simulink model "EurlerDynJointVerify"  (Simulink 7.6)
settings: Solver=ode45  StartTime=0.0  StopTime=10  RelTol=1e-3
InitFcn:
  | eval('Config')
  | %eval('EfortConfig')
values from neighbouring files (symbols this model uses):
  a2 = 0    [Config.m]    (also in CtrPlatformCfg.m)
  a3 = 0    [Config.m]    (also in CtrPlatformCfg.m)
  a4 = 0    [Config.m]    (also in CtrPlatformCfg.m)
  a5 = 90    [Config.m]    (also in CtrPlatformCfg.m)
  a6 = 0    [Config.m]    (also in CtrPlatformCfg.m)
  Cen_EU = Cen    [DynEulerTest.m]
  DH_EU = [266     300     0       0       1016     0      174 ... (first row only)    [DynEulerTest.m]
  freq = tvel/radius    (= 1)    [Config.m]    (also in CtrPlatformCfg.m)
  Ft_EU = [0;0;0;0;0;0]    [DynEulerTest.m]
  Ie_EU = [Ie1;Ie2;Ie3;Ie4;Ie5;Ie6]    [DynEulerTest.m]
  init_Endx = gd_init(1,4)    [Config.m]    (also in CtrPlatformCfg.m)
  init_Endy = gd_init(2,4)    [Config.m]    (also in CtrPlatformCfg.m)
  init_Endz = gd_init(3,4)    [Config.m]    (also in CtrPlatformCfg.m)
  init_Rot = gd_init(1:3,1:3)    [Config.m]    (also in CtrPlatformCfg.m)
  L = [l1 l2 l3 l4 l5 l6 l7 l8 l9]    [Config.m]    (also in CtrPlatformCfg.m)
  Ma_EU = Ma    [DynEulerTest.m]
  tvel = 120    [Config.m]    (also in CtrPlatformCfg.m)
undefined symbols (not defined in the file or in its folder): a1, Cen_Min, DH_Min, Ft_Min, Ie_Min, Ma_Min
libraries: mblibv1 x41, simulink x9
(part 3 of 3)

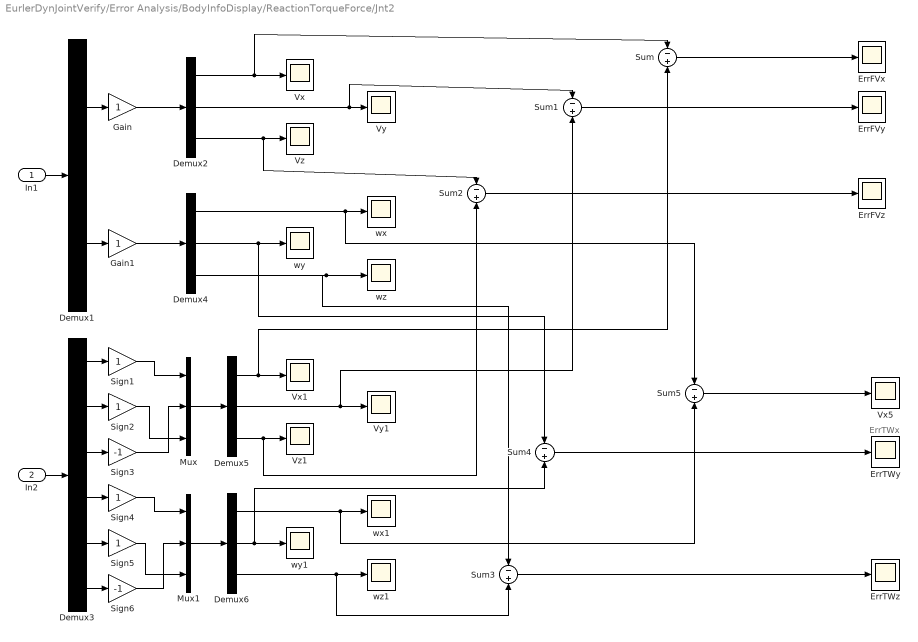
== system EurlerDynJointVerify/Error Analysis/BodyInfoDisplay/ReactionTorqueForce/Jnt2 ==
  note: ErrTWx
  In1 : Inport
  In2 : Inport  Port=2
  Demux1 : Demux  Outputs=2
  Demux{2,4..6} (4 alike) : Demux  Outputs=3
  Demux3 : Demux  Outputs=6
  ErrFVx : Scope
      settings: TimeRange=10  YMin=-3e-017  YMax=4e-017  SaveName=ScopeData51
  ErrFVy : Scope
      settings: TimeRange=10  YMin=-3e-017  YMax=4e-017  SaveName=ScopeData52
  ErrFVz : Scope
      settings: TimeRange=10  YMin=-3e-017  YMax=4e-017  SaveName=ScopeData53
  ErrTWy : Scope
      settings: TimeRange=10  YMin=-3e-017  YMax=4e-017  SaveName=ScopeData56
  ErrTWz : Scope
      settings: TimeRange=3  YMin=-1.5e-014  YMax=1.5e-014  SaveName=ScopeData68
  Gain : Gain
  Gain1 : Gain
  Mux : Mux  Inputs=3
  Mux1 : Mux  Inputs=3
  Sign{1..2,4..5} (4 alike) : Gain
  Sign3 : Gain  Gain=-1
  Sign6 : Gain  Gain=-1
  Sum{,1..5} (6 alike) : Sum  Inputs=-|+
  Vx : Scope
      settings: TimeRange=10  YMin=-3e-017  YMax=4e-017  SaveName=ScopeData40
  Vx1 : Scope
      settings: TimeRange=10  YMin=-3e-017  YMax=4e-017  SaveName=ScopeData45
  Vx5 : Scope
      settings: TimeRange=10  YMin=-3e-017  YMax=4e-017  SaveName=ScopeData54
  Vy : Scope
      settings: TimeRange=10  YMin=-3e-017  YMax=4e-017  SaveName=ScopeData39
  Vy1 : Scope
      settings: TimeRange=10  YMin=-3e-017  YMax=4e-017  SaveName=ScopeData46
  Vz : Scope
      settings: TimeRange=10  YMin=-3e-017  YMax=4e-017  SaveName=ScopeData41
  Vz1 : Scope
      settings: TimeRange=10  YMin=-3e-017  YMax=4e-017  SaveName=ScopeData47
  wx : Scope
      settings: TimeRange=3  YMin=-125  YMax=125  SaveName=ScopeData42
  wx1 : Scope
      settings: TimeRange=3  YMin=-125  YMax=125  SaveName=ScopeData48
  wy : Scope
      settings: TimeRange=10  YMin=-3e-017  YMax=4e-017  SaveName=ScopeData43
  wy1 : Scope
      settings: TimeRange=10  YMin=-3e-017  YMax=4e-017  SaveName=ScopeData49
  wz : Scope
      settings: TimeRange=10  YMin=-3e-017  YMax=4e-017  SaveName=ScopeData44
  wz1 : Scope
      settings: TimeRange=10  YMin=-3e-017  YMax=4e-017  SaveName=ScopeData50
  wires:
  Sign4/1 -> Mux1/1
  Sign1/1 -> Mux/1
  Demux3/6 -> Sign6/1
  Demux3/5 -> Sign5/1
  Demux3/4 -> Sign4/1
  Demux3/3 -> Sign3/1
  Demux3/2 -> Sign2/1
  Demux3/1 -> Sign1/1
  Mux1/1 -> Demux6/1
  Mux/1 -> Demux5/1
  Sum/1 -> ErrFVx/1
  Sum1/1 -> ErrFVy/1
  Sum2/1 -> ErrFVz/1
  Sum3/1 -> ErrTWz/1
  Sum4/1 -> ErrTWy/1
  Sum5/1 -> Vx5/1
  In2/1 -> Demux3/1
  Demux6/3 -> Sum3/2, wz1/1
  Demux6/2 -> Sum4/2, wy1/1
  Demux6/1 -> Sum5/2, wx1/1
  Demux5/3 -> Sum2/2, Vz1/1
  Demux5/2 -> Sum1/2, Vy1/1
  Demux5/1 -> Sum/2, Vx1/1
  In1/1 -> Demux1/1
  Demux4/3 -> Sum3/1, wz/1
  Demux4/2 -> Sum4/1, wy/1
  Demux4/1 -> Sum5/1, wx/1
  Demux2/3 -> Sum2/1, Vz/1
  Demux2/2 -> Sum1/1, Vy/1
  Demux2/1 -> Sum/1, Vx/1
  Gain1/1 -> Demux4/1
  Gain/1 -> Demux2/1
  Demux1/2 -> Gain1/1
  Demux1/1 -> Gain/1
  Sign3/1 -> Mux/2
  Sign2/1 -> Mux/3
  Sign6/1 -> Mux1/2
  Sign5/1 -> Mux1/3

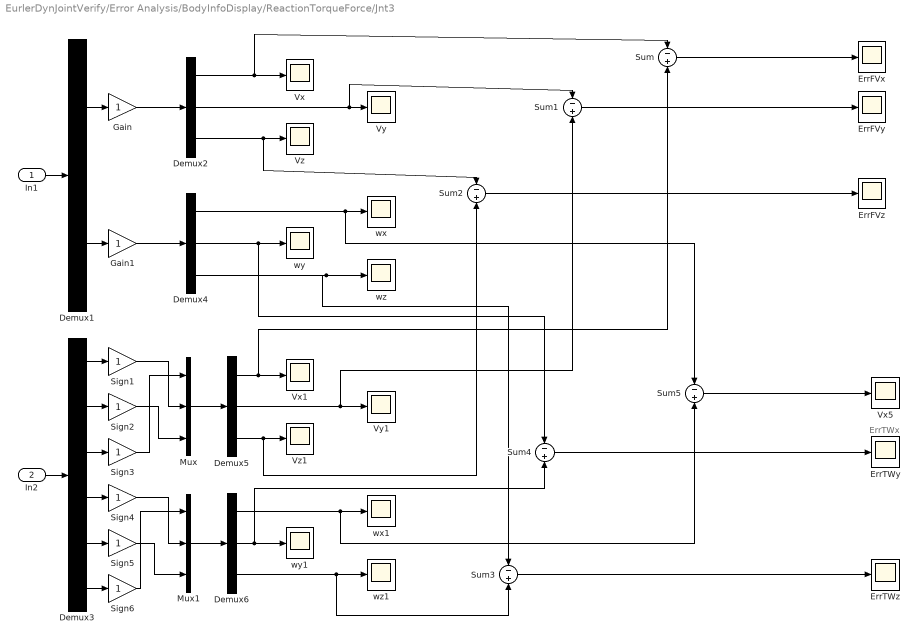
== system EurlerDynJointVerify/Error Analysis/BodyInfoDisplay/ReactionTorqueForce/Jnt3 ==
  note: ErrTWx
  In1 : Inport
  In2 : Inport  Port=2
  Demux1 : Demux  Outputs=2
  Demux{2,4..6} (4 alike) : Demux  Outputs=3
  Demux3 : Demux  Outputs=6
  ErrFVx : Scope
      settings: TimeRange=10  YMin=-3e-017  YMax=4e-017  SaveName=ScopeData51
  ErrFVy : Scope
      settings: TimeRange=10  YMin=-3e-017  YMax=4e-017  SaveName=ScopeData52
  ErrFVz : Scope
      settings: TimeRange=10  YMin=-3e-017  YMax=4e-017  SaveName=ScopeData53
  ErrTWy : Scope
      settings: TimeRange=10  YMin=-3e-017  YMax=4e-017  SaveName=ScopeData56
  ErrTWz : Scope
      settings: TimeRange=10  YMin=-3e-017  YMax=4e-017  SaveName=ScopeData68
  Gain : Gain
  Gain1 : Gain
  Mux : Mux  Inputs=3
  Mux1 : Mux  Inputs=3
  Sign{1..6} (6 alike) : Gain
  Sum{,1..5} (6 alike) : Sum  Inputs=-|+
  Vx : Scope
      settings: TimeRange=10  YMin=-3e-017  YMax=4e-017  SaveName=ScopeData40
  Vx1 : Scope
      settings: TimeRange=10  YMin=-3e-017  YMax=4e-017  SaveName=ScopeData45
  Vx5 : Scope
      settings: TimeRange=10  YMin=-3e-017  YMax=4e-017  SaveName=ScopeData54
  Vy : Scope
      settings: TimeRange=10  YMin=-3e-017  YMax=4e-017  SaveName=ScopeData39
  Vy1 : Scope
      settings: TimeRange=10  YMin=-3e-017  YMax=4e-017  SaveName=ScopeData46
  Vz : Scope
      settings: TimeRange=10  YMin=-3e-017  YMax=4e-017  SaveName=ScopeData41
  Vz1 : Scope
      settings: TimeRange=10  YMin=-3e-017  YMax=4e-017  SaveName=ScopeData47
  wx : Scope
      settings: TimeRange=3  YMin=-125  YMax=125  SaveName=ScopeData42
  wx1 : Scope
      settings: TimeRange=3  YMin=-125  YMax=125  SaveName=ScopeData48
  wy : Scope
      settings: TimeRange=10  YMin=-3e-017  YMax=4e-017  SaveName=ScopeData43
  wy1 : Scope
      settings: TimeRange=10  YMin=-3e-017  YMax=4e-017  SaveName=ScopeData49
  wz : Scope
      settings: TimeRange=10  YMin=-3e-017  YMax=4e-017  SaveName=ScopeData44
  wz1 : Scope
      settings: TimeRange=10  YMin=-3e-017  YMax=4e-017  SaveName=ScopeData50
  wires:
  Demux1/1 -> Gain/1
  Demux1/2 -> Gain1/1
  Gain/1 -> Demux2/1
  Gain1/1 -> Demux4/1
  Demux2/1 -> Vx/1, Sum/1
  Demux2/2 -> Vy/1, Sum1/1
  Demux2/3 -> Vz/1, Sum2/1
  Demux4/1 -> wx/1, Sum5/1
  Demux4/2 -> wy/1, Sum4/1
  Demux4/3 -> wz/1, Sum3/1
  In1/1 -> Demux1/1
  Demux5/1 -> Vx1/1, Sum/2
  Demux5/2 -> Vy1/1, Sum1/2
  Demux5/3 -> Vz1/1, Sum2/2
  Demux6/1 -> wx1/1, Sum5/2
  Demux6/2 -> wy1/1, Sum4/2
  Demux6/3 -> wz1/1, Sum3/2
  In2/1 -> Demux3/1
  Sum5/1 -> Vx5/1
  Sum4/1 -> ErrTWy/1
  Sum3/1 -> ErrTWz/1
  Sum2/1 -> ErrFVz/1
  Sum1/1 -> ErrFVy/1
  Sum/1 -> ErrFVx/1
  Mux/1 -> Demux5/1
  Mux1/1 -> Demux6/1
  Demux3/1 -> Sign1/1
  Demux3/2 -> Sign2/1
  Demux3/3 -> Sign3/1
  Demux3/4 -> Sign4/1
  Demux3/5 -> Sign5/1
  Demux3/6 -> Sign6/1
  Sign1/1 -> Mux/2
  Sign2/1 -> Mux/3
  Sign3/1 -> Mux/1
  Sign4/1 -> Mux1/2
  Sign5/1 -> Mux1/3
  Sign6/1 -> Mux1/1

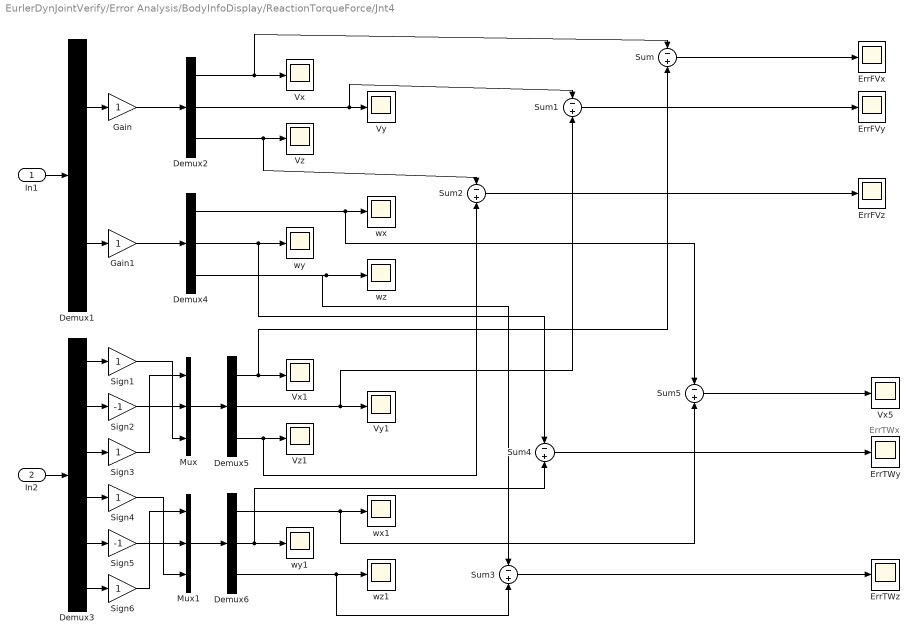
== system EurlerDynJointVerify/Error Analysis/BodyInfoDisplay/ReactionTorqueForce/Jnt4 ==
  note: ErrTWx
  In1 : Inport
  In2 : Inport  Port=2
  Demux1 : Demux  Outputs=2
  Demux{2,4..6} (4 alike) : Demux  Outputs=3
  Demux3 : Demux  Outputs=6
  ErrFVx : Scope
      settings: TimeRange=10  YMin=-3e-017  YMax=4e-017  SaveName=ScopeData51
  ErrFVy : Scope
      settings: TimeRange=10  YMin=-3e-017  YMax=4e-017  SaveName=ScopeData52
  ErrFVz : Scope
      settings: TimeRange=10  YMin=-3e-017  YMax=4e-017  SaveName=ScopeData53
  ErrTWy : Scope
      settings: TimeRange=10  YMin=-3e-017  YMax=4e-017  SaveName=ScopeData56
  ErrTWz : Scope
      settings: TimeRange=10  YMin=-3e-017  YMax=4e-017  SaveName=ScopeData68
  Gain : Gain
  Gain1 : Gain
  Mux : Mux  Inputs=3
  Mux1 : Mux  Inputs=3
  Sign{1,3..4,6} (4 alike) : Gain
  Sign2 : Gain  Gain=-1
  Sign5 : Gain  Gain=-1
  Sum{,1..5} (6 alike) : Sum  Inputs=-|+
  Vx : Scope
      settings: TimeRange=10  YMin=-3e-017  YMax=4e-017  SaveName=ScopeData40
  Vx1 : Scope
      settings: TimeRange=10  YMin=-3e-017  YMax=4e-017  SaveName=ScopeData45
  Vx5 : Scope
      settings: TimeRange=10  YMin=-3e-017  YMax=4e-017  SaveName=ScopeData54
  Vy : Scope
      settings: TimeRange=10  YMin=-3e-017  YMax=4e-017  SaveName=ScopeData39
  Vy1 : Scope
      settings: TimeRange=10  YMin=-3e-017  YMax=4e-017  SaveName=ScopeData46
  Vz : Scope
      settings: TimeRange=10  YMin=-3e-017  YMax=4e-017  SaveName=ScopeData41
  Vz1 : Scope
      settings: TimeRange=10  YMin=-3e-017  YMax=4e-017  SaveName=ScopeData47
  wx : Scope
      settings: TimeRange=3  YMin=-125  YMax=125  SaveName=ScopeData42
  wx1 : Scope
      settings: TimeRange=3  YMin=-125  YMax=125  SaveName=ScopeData48
  wy : Scope
      settings: TimeRange=10  YMin=-3e-017  YMax=4e-017  SaveName=ScopeData43
  wy1 : Scope
      settings: TimeRange=10  YMin=-3e-017  YMax=4e-017  SaveName=ScopeData49
  wz : Scope
      settings: TimeRange=10  YMin=-3e-017  YMax=4e-017  SaveName=ScopeData44
  wz1 : Scope
      settings: TimeRange=10  YMin=-3e-017  YMax=4e-017  SaveName=ScopeData50
  wires:
  Demux3/6 -> Sign6/1
  Demux3/5 -> Sign5/1
  Demux3/4 -> Sign4/1
  Demux3/3 -> Sign3/1
  Demux3/2 -> Sign2/1
  Demux3/1 -> Sign1/1
  Mux1/1 -> Demux6/1
  Mux/1 -> Demux5/1
  Sum/1 -> ErrFVx/1
  Sum1/1 -> ErrFVy/1
  Sum2/1 -> ErrFVz/1
  Sum3/1 -> ErrTWz/1
  Sum4/1 -> ErrTWy/1
  Sum5/1 -> Vx5/1
  In2/1 -> Demux3/1
  Demux6/3 -> Sum3/2, wz1/1
  Demux6/2 -> Sum4/2, wy1/1
  Demux6/1 -> Sum5/2, wx1/1
  Demux5/3 -> Sum2/2, Vz1/1
  Demux5/2 -> Sum1/2, Vy1/1
  Demux5/1 -> Sum/2, Vx1/1
  In1/1 -> Demux1/1
  Demux4/3 -> Sum3/1, wz/1
  Demux4/2 -> Sum4/1, wy/1
  Demux4/1 -> Sum5/1, wx/1
  Demux2/3 -> Sum2/1, Vz/1
  Demux2/2 -> Sum1/1, Vy/1
  Demux2/1 -> Sum/1, Vx/1
  Gain1/1 -> Demux4/1
  Gain/1 -> Demux2/1
  Demux1/2 -> Gain1/1
  Demux1/1 -> Gain/1
  Sign1/1 -> Mux/3
  Sign2/1 -> Mux/2
  Sign3/1 -> Mux/1
  Sign4/1 -> Mux1/3
  Sign5/1 -> Mux1/2
  Sign6/1 -> Mux1/1

== system EurlerDynJointVerify/Error Analysis/BodyInfoDisplay/ReactionTorqueForce/Jnt5 ==
  note: ErrTWx
  In1 : Inport
  In2 : Inport  Port=2
  Demux1 : Demux  Outputs=2
  Demux{2,4..6} (4 alike) : Demux  Outputs=3
  Demux3 : Demux  Outputs=6
  ErrFVx : Scope
      settings: TimeRange=10  YMin=-3e-017  YMax=4e-017  SaveName=ScopeData51
  ErrFVy : Scope
      settings: TimeRange=10  YMin=-3e-017  YMax=4e-017  SaveName=ScopeData52
  ErrFVz : Scope
      settings: TimeRange=10  YMin=-3e-017  YMax=4e-017  SaveName=ScopeData53
  ErrTWy : Scope
      settings: TimeRange=10  YMin=-3e-017  YMax=4e-017  SaveName=ScopeData56
  ErrTWz : Scope
      settings: TimeRange=10  YMin=-3e-017  YMax=4e-017  SaveName=ScopeData68
  Gain : Gain
  Gain1 : Gain
  Mux : Mux  Inputs=3
  Mux1 : Mux  Inputs=3
  Sign{1,3..4,6} (4 alike) : Gain  Gain=-1
  Sign2 : Gain
  Sign5 : Gain
  Sum{,1..5} (6 alike) : Sum  Inputs=-|+
  Vx : Scope
      settings: TimeRange=10  YMin=-3e-017  YMax=4e-017  SaveName=ScopeData40
  Vx1 : Scope
      settings: TimeRange=10  YMin=-3e-017  YMax=4e-017  SaveName=ScopeData45
  Vx5 : Scope
      settings: TimeRange=10  YMin=-3e-017  YMax=4e-017  SaveName=ScopeData54
  Vy : Scope
      settings: TimeRange=10  YMin=-3e-017  YMax=4e-017  SaveName=ScopeData39
  Vy1 : Scope
      settings: TimeRange=10  YMin=-3e-017  YMax=4e-017  SaveName=ScopeData46
  Vz : Scope
      settings: TimeRange=10  YMin=-3e-017  YMax=4e-017  SaveName=ScopeData41
  Vz1 : Scope
      settings: TimeRange=10  YMin=-3e-017  YMax=4e-017  SaveName=ScopeData47
  wx : Scope
      settings: TimeRange=3  YMin=-125  YMax=125  SaveName=ScopeData42
  wx1 : Scope
      settings: TimeRange=3  YMin=-125  YMax=125  SaveName=ScopeData48
  wy : Scope
      settings: TimeRange=10  YMin=-3e-017  YMax=4e-017  SaveName=ScopeData43
  wy1 : Scope
      settings: TimeRange=10  YMin=-3e-017  YMax=4e-017  SaveName=ScopeData49
  wz : Scope
      settings: TimeRange=10  YMin=-3e-017  YMax=4e-017  SaveName=ScopeData44
  wz1 : Scope
      settings: TimeRange=10  YMin=-3e-017  YMax=4e-017  SaveName=ScopeData50
  wires:
  Demux1/1 -> Gain/1
  Demux1/2 -> Gain1/1
  Gain/1 -> Demux2/1
  Gain1/1 -> Demux4/1
  Demux2/1 -> Vx/1, Sum/1
  Demux2/2 -> Vy/1, Sum1/1
  Demux2/3 -> Vz/1, Sum2/1
  Demux4/1 -> wx/1, Sum5/1
  Demux4/2 -> wy/1, Sum4/1
  Demux4/3 -> wz/1, Sum3/1
  In1/1 -> Demux1/1
  Demux5/1 -> Vx1/1, Sum/2
  Demux5/2 -> Vy1/1, Sum1/2
  Demux5/3 -> Vz1/1, Sum2/2
  Demux6/1 -> wx1/1, Sum5/2
  Demux6/2 -> wy1/1, Sum4/2
  Demux6/3 -> wz1/1, Sum3/2
  In2/1 -> Demux3/1
  Sum5/1 -> Vx5/1
  Sum4/1 -> ErrTWy/1
  Sum3/1 -> ErrTWz/1
  Sum2/1 -> ErrFVz/1
  Sum1/1 -> ErrFVy/1
  Sum/1 -> ErrFVx/1
  Mux/1 -> Demux5/1
  Mux1/1 -> Demux6/1
  Demux3/1 -> Sign1/1
  Demux3/2 -> Sign2/1
  Demux3/3 -> Sign3/1
  Demux3/4 -> Sign4/1
  Demux3/5 -> Sign5/1
  Demux3/6 -> Sign6/1
  Sign1/1 -> Mux/2
  Sign2/1 -> Mux/3
  Sign3/1 -> Mux/1
  Sign4/1 -> Mux1/2
  Sign5/1 -> Mux1/3
  Sign6/1 -> Mux1/1

== system EurlerDynJointVerify/Error Analysis/BodyInfoDisplay/ReactionTorqueForce/Jnt6 ==
  note: ErrTWx
  In1 : Inport
  In2 : Inport  Port=2
  Demux1 : Demux  Outputs=2
  Demux{2,4..6} (4 alike) : Demux  Outputs=3
  Demux3 : Demux  Outputs=6
  ErrFVx : Scope
      settings: TimeRange=10  YMin=-3e-017  YMax=4e-017  SaveName=ScopeData51
  ErrFVy : Scope
      settings: TimeRange=10  YMin=-3e-017  YMax=4e-017  SaveName=ScopeData52
  ErrFVz : Scope
      settings: TimeRange=10  YMin=-3e-017  YMax=4e-017  SaveName=ScopeData53
  ErrTWy : Scope
      settings: TimeRange=10  YMin=-3e-017  YMax=4e-017  SaveName=ScopeData56
  ErrTWz : Scope
      settings: TimeRange=10  YMin=-3e-017  YMax=4e-017  SaveName=ScopeData68
  Gain : Gain
  Gain1 : Gain
  Mux : Mux  Inputs=3
  Mux1 : Mux  Inputs=3
  Sign{1,3..4,6} (4 alike) : Gain
  Sign2 : Gain  Gain=-1
  Sign5 : Gain  Gain=-1
  Sum{,1..5} (6 alike) : Sum  Inputs=-|+
  Vx : Scope
      settings: TimeRange=10  YMin=-3e-017  YMax=4e-017  SaveName=ScopeData40
  Vx1 : Scope
      settings: TimeRange=10  YMin=-3e-017  YMax=4e-017  SaveName=ScopeData45
  Vx5 : Scope
      settings: TimeRange=10  YMin=-3e-017  YMax=4e-017  SaveName=ScopeData54
  Vy : Scope
      settings: TimeRange=10  YMin=-3e-017  YMax=4e-017  SaveName=ScopeData39
  Vy1 : Scope
      settings: TimeRange=10  YMin=-3e-017  YMax=4e-017  SaveName=ScopeData46
  Vz : Scope
      settings: TimeRange=10  YMin=-3e-017  YMax=4e-017  SaveName=ScopeData41
  Vz1 : Scope
      settings: TimeRange=10  YMin=-3e-017  YMax=4e-017  SaveName=ScopeData47
  wx : Scope
      settings: TimeRange=3  YMin=-125  YMax=125  SaveName=ScopeData42
  wx1 : Scope
      settings: TimeRange=3  YMin=-125  YMax=125  SaveName=ScopeData48
  wy : Scope
      settings: TimeRange=10  YMin=-3e-017  YMax=4e-017  SaveName=ScopeData43
  wy1 : Scope
      settings: TimeRange=10  YMin=-3e-017  YMax=4e-017  SaveName=ScopeData49
  wz : Scope
      settings: TimeRange=10  YMin=-3e-017  YMax=4e-017  SaveName=ScopeData44
  wz1 : Scope
      settings: TimeRange=10  YMin=-3e-017  YMax=4e-017  SaveName=ScopeData50
  wires:
  Demux3/6 -> Sign6/1
  Demux3/5 -> Sign5/1
  Demux3/4 -> Sign4/1
  Demux3/3 -> Sign3/1
  Demux3/2 -> Sign2/1
  Demux3/1 -> Sign1/1
  Mux1/1 -> Demux6/1
  Mux/1 -> Demux5/1
  Sum/1 -> ErrFVx/1
  Sum1/1 -> ErrFVy/1
  Sum2/1 -> ErrFVz/1
  Sum3/1 -> ErrTWz/1
  Sum4/1 -> ErrTWy/1
  Sum5/1 -> Vx5/1
  In2/1 -> Demux3/1
  Demux6/3 -> Sum3/2, wz1/1
  Demux6/2 -> Sum4/2, wy1/1
  Demux6/1 -> Sum5/2, wx1/1
  Demux5/3 -> Sum2/2, Vz1/1
  Demux5/2 -> Sum1/2, Vy1/1
  Demux5/1 -> Sum/2, Vx1/1
  In1/1 -> Demux1/1
  Demux4/3 -> Sum3/1, wz/1
  Demux4/2 -> Sum4/1, wy/1
  Demux4/1 -> Sum5/1, wx/1
  Demux2/3 -> Sum2/1, Vz/1
  Demux2/2 -> Sum1/1, Vy/1
  Demux2/1 -> Sum/1, Vx/1
  Gain1/1 -> Demux4/1
  Gain/1 -> Demux2/1
  Demux1/2 -> Gain1/1
  Demux1/1 -> Gain/1
  Sign1/1 -> Mux/3
  Sign2/1 -> Mux/2
  Sign3/1 -> Mux/1
  Sign4/1 -> Mux1/3
  Sign5/1 -> Mux1/2
  Sign6/1 -> Mux1/1

== system EurlerDynJointVerify/Error Analysis/BodyInfoDisplay/Vel/Jnt1 ==
  note: ErrWx
  In1 : Inport
  In2 : Inport  Port=2
  Demux1 : Demux  Outputs=2
  Demux{2,4..6} (4 alike) : Demux  Outputs=3
  Demux3 : Demux  Outputs=6
  ErrVx : Scope
      settings: TimeRange=10  YMin=-3e-017  YMax=4e-017  SaveName=ScopeData51
  ErrVy : Scope
      settings: TimeRange=10  YMin=-3e-017  YMax=4e-017  SaveName=ScopeData52
  ErrVz : Scope
      settings: TimeRange=10  YMin=-3e-017  YMax=4e-017  SaveName=ScopeData53
  ErrWy : Scope
      settings: TimeRange=10  YMin=-3e-017  YMax=4e-017  SaveName=ScopeData56
  ErrWz : Scope
      settings: TimeRange=10  YMin=-3e-017  YMax=4e-017  SaveName=ScopeData68
  Gain : Gain  Gain=1000
  Gain1 : Gain  Gain=180/pi
  Mux : Mux  Inputs=3
  Mux1 : Mux  Inputs=3
  Sign{1..6} (6 alike) : Gain
  Sum{,1..5} (6 alike) : Sum  Inputs=-|+
  Vx : Scope
      settings: TimeRange=10  YMin=-3e-017  YMax=4e-017  SaveName=ScopeData40
  Vx1 : Scope
      settings: TimeRange=10  YMin=-3e-017  YMax=4e-017  SaveName=ScopeData45
  Vx5 : Scope
      settings: TimeRange=10  YMin=-3e-017  YMax=4e-017  SaveName=ScopeData54
  Vy : Scope
      settings: TimeRange=10  YMin=-3e-017  YMax=4e-017  SaveName=ScopeData39
  Vy1 : Scope
      settings: TimeRange=10  YMin=-3e-017  YMax=4e-017  SaveName=ScopeData46
  Vz : Scope
      settings: TimeRange=10  YMin=-3e-017  YMax=4e-017  SaveName=ScopeData41
  Vz1 : Scope
      settings: TimeRange=10  YMin=-3e-017  YMax=4e-017  SaveName=ScopeData47
  wx : Scope
      settings: TimeRange=3  YMin=-125  YMax=125  SaveName=ScopeData42
  wx1 : Scope
      settings: TimeRange=3  YMin=-125  YMax=125  SaveName=ScopeData48
  wy : Scope
      settings: TimeRange=10  YMin=-3e-017  YMax=4e-017  SaveName=ScopeData43
  wy1 : Scope
      settings: TimeRange=10  YMin=-3e-017  YMax=4e-017  SaveName=ScopeData49
  wz : Scope
      settings: TimeRange=10  YMin=-3e-017  YMax=4e-017  SaveName=ScopeData44
  wz1 : Scope
      settings: TimeRange=10  YMin=-3e-017  YMax=4e-017  SaveName=ScopeData50
  wires:
  Demux1/1 -> Gain/1
  Demux1/2 -> Gain1/1
  Gain/1 -> Demux2/1
  Gain1/1 -> Demux4/1
  Demux2/1 -> Vx/1, Sum/1
  Demux2/2 -> Vy/1, Sum1/1
  Demux2/3 -> Vz/1, Sum2/1
  Demux4/1 -> wx/1, Sum5/1
  Demux4/2 -> wy/1, Sum4/1
  Demux4/3 -> wz/1, Sum3/1
  In1/1 -> Demux1/1
  Demux5/1 -> Vx1/1, Sum/2
  Demux5/2 -> Vy1/1, Sum1/2
  Demux5/3 -> Vz1/1, Sum2/2
  Demux6/1 -> wx1/1, Sum5/2
  Demux6/2 -> wy1/1, Sum4/2
  Demux6/3 -> wz1/1, Sum3/2
  In2/1 -> Demux3/1
  Sum5/1 -> Vx5/1
  Sum4/1 -> ErrWy/1
  Sum3/1 -> ErrWz/1
  Sum2/1 -> ErrVz/1
  Sum1/1 -> ErrVy/1
  Sum/1 -> ErrVx/1
  Mux/1 -> Demux5/1
  Mux1/1 -> Demux6/1
  Demux3/1 -> Sign1/1
  Demux3/2 -> Sign2/1
  Demux3/3 -> Sign3/1
  Demux3/4 -> Sign4/1
  Demux3/5 -> Sign5/1
  Demux3/6 -> Sign6/1
  Sign1/1 -> Mux/1
  Sign2/1 -> Mux/2
  Sign3/1 -> Mux/3
  Sign4/1 -> Mux1/1
  Sign5/1 -> Mux1/2
  Sign6/1 -> Mux1/3

== system EurlerDynJointVerify/Error Analysis/BodyInfoDisplay/Vel/Jnt2 ==
  note: ErrWx
  In1 : Inport
  In2 : Inport  Port=2
  Demux1 : Demux  Outputs=2
  Demux{2,4..6} (4 alike) : Demux  Outputs=3
  Demux3 : Demux  Outputs=6
  ErrVx : Scope
      settings: TimeRange=10  YMin=-3e-017  YMax=4e-017  SaveName=ScopeData51
  ErrVy : Scope
      settings: TimeRange=10  YMin=-3e-017  YMax=4e-017  SaveName=ScopeData52
  ErrVz : Scope
      settings: TimeRange=10  YMin=-3e-017  YMax=4e-017  SaveName=ScopeData53
  ErrWy : Scope
      settings: TimeRange=10  YMin=-3e-017  YMax=4e-017  SaveName=ScopeData56
  ErrWz : Scope
      settings: TimeRange=3  YMin=-1.5e-014  YMax=1.5e-014  SaveName=ScopeData68
  Gain : Gain  Gain=1000
  Gain1 : Gain  Gain=180/pi
  Mux : Mux  Inputs=3
  Mux1 : Mux  Inputs=3
  Sign{1..2,4..5} (4 alike) : Gain
  Sign3 : Gain  Gain=-1
  Sign6 : Gain  Gain=-1
  Sum{,1..5} (6 alike) : Sum  Inputs=-|+
  Vx : Scope
      settings: TimeRange=10  YMin=-3e-017  YMax=4e-017  SaveName=ScopeData40
  Vx1 : Scope
      settings: TimeRange=10  YMin=-3e-017  YMax=4e-017  SaveName=ScopeData45
  Vx5 : Scope
      settings: TimeRange=10  YMin=-3e-017  YMax=4e-017  SaveName=ScopeData54
  Vy : Scope
      settings: TimeRange=10  YMin=-3e-017  YMax=4e-017  SaveName=ScopeData39
  Vy1 : Scope
      settings: TimeRange=10  YMin=-3e-017  YMax=4e-017  SaveName=ScopeData46
  Vz : Scope
      settings: TimeRange=10  YMin=-3e-017  YMax=4e-017  SaveName=ScopeData41
  Vz1 : Scope
      settings: TimeRange=10  YMin=-3e-017  YMax=4e-017  SaveName=ScopeData47
  wx : Scope
      settings: TimeRange=3  YMin=-125  YMax=125  SaveName=ScopeData42
  wx1 : Scope
      settings: TimeRange=3  YMin=-125  YMax=125  SaveName=ScopeData48
  wy : Scope
      settings: TimeRange=10  YMin=-3e-017  YMax=4e-017  SaveName=ScopeData43
  wy1 : Scope
      settings: TimeRange=10  YMin=-3e-017  YMax=4e-017  SaveName=ScopeData49
  wz : Scope
      settings: TimeRange=10  YMin=-3e-017  YMax=4e-017  SaveName=ScopeData44
  wz1 : Scope
      settings: TimeRange=10  YMin=-3e-017  YMax=4e-017  SaveName=ScopeData50
  wires:
  Sign4/1 -> Mux1/1
  Sign1/1 -> Mux/1
  Demux3/6 -> Sign6/1
  Demux3/5 -> Sign5/1
  Demux3/4 -> Sign4/1
  Demux3/3 -> Sign3/1
  Demux3/2 -> Sign2/1
  Demux3/1 -> Sign1/1
  Mux1/1 -> Demux6/1
  Mux/1 -> Demux5/1
  Sum/1 -> ErrVx/1
  Sum1/1 -> ErrVy/1
  Sum2/1 -> ErrVz/1
  Sum3/1 -> ErrWz/1
  Sum4/1 -> ErrWy/1
  Sum5/1 -> Vx5/1
  In2/1 -> Demux3/1
  Demux6/3 -> Sum3/2, wz1/1
  Demux6/2 -> Sum4/2, wy1/1
  Demux6/1 -> Sum5/2, wx1/1
  Demux5/3 -> Sum2/2, Vz1/1
  Demux5/2 -> Sum1/2, Vy1/1
  Demux5/1 -> Sum/2, Vx1/1
  In1/1 -> Demux1/1
  Demux4/3 -> Sum3/1, wz/1
  Demux4/2 -> Sum4/1, wy/1
  Demux4/1 -> Sum5/1, wx/1
  Demux2/3 -> Sum2/1, Vz/1
  Demux2/2 -> Sum1/1, Vy/1
  Demux2/1 -> Sum/1, Vx/1
  Gain1/1 -> Demux4/1
  Gain/1 -> Demux2/1
  Demux1/2 -> Gain1/1
  Demux1/1 -> Gain/1
  Sign3/1 -> Mux/2
  Sign2/1 -> Mux/3
  Sign6/1 -> Mux1/2
  Sign5/1 -> Mux1/3

== system EurlerDynJointVerify/Error Analysis/BodyInfoDisplay/Vel/Jnt3 ==
  note: ErrWx
  In1 : Inport
  In2 : Inport  Port=2
  Demux1 : Demux  Outputs=2
  Demux{2,4..6} (4 alike) : Demux  Outputs=3
  Demux3 : Demux  Outputs=6
  ErrVx : Scope
      settings: TimeRange=10  YMin=-3e-017  YMax=4e-017  SaveName=ScopeData51
  ErrVy : Scope
      settings: TimeRange=10  YMin=-3e-017  YMax=4e-017  SaveName=ScopeData52
  ErrVz : Scope
      settings: TimeRange=10  YMin=-3e-017  YMax=4e-017  SaveName=ScopeData53
  ErrWy : Scope
      settings: TimeRange=10  YMin=-3e-017  YMax=4e-017  SaveName=ScopeData56
  ErrWz : Scope
      settings: TimeRange=10  YMin=-3e-017  YMax=4e-017  SaveName=ScopeData68
  Gain : Gain  Gain=1000
  Gain1 : Gain  Gain=180/pi
  Mux : Mux  Inputs=3
  Mux1 : Mux  Inputs=3
  Sign{1..6} (6 alike) : Gain
  Sum{,1..5} (6 alike) : Sum  Inputs=-|+
  Vx : Scope
      settings: TimeRange=10  YMin=-3e-017  YMax=4e-017  SaveName=ScopeData40
  Vx1 : Scope
      settings: TimeRange=10  YMin=-3e-017  YMax=4e-017  SaveName=ScopeData45
  Vx5 : Scope
      settings: TimeRange=10  YMin=-3e-017  YMax=4e-017  SaveName=ScopeData54
  Vy : Scope
      settings: TimeRange=10  YMin=-3e-017  YMax=4e-017  SaveName=ScopeData39
  Vy1 : Scope
      settings: TimeRange=10  YMin=-3e-017  YMax=4e-017  SaveName=ScopeData46
  Vz : Scope
      settings: TimeRange=10  YMin=-3e-017  YMax=4e-017  SaveName=ScopeData41
  Vz1 : Scope
      settings: TimeRange=10  YMin=-3e-017  YMax=4e-017  SaveName=ScopeData47
  wx : Scope
      settings: TimeRange=3  YMin=-125  YMax=125  SaveName=ScopeData42
  wx1 : Scope
      settings: TimeRange=3  YMin=-125  YMax=125  SaveName=ScopeData48
  wy : Scope
      settings: TimeRange=10  YMin=-3e-017  YMax=4e-017  SaveName=ScopeData43
  wy1 : Scope
      settings: TimeRange=10  YMin=-3e-017  YMax=4e-017  SaveName=ScopeData49
  wz : Scope
      settings: TimeRange=10  YMin=-3e-017  YMax=4e-017  SaveName=ScopeData44
  wz1 : Scope
      settings: TimeRange=10  YMin=-3e-017  YMax=4e-017  SaveName=ScopeData50
  wires:
  Demux1/1 -> Gain/1
  Demux1/2 -> Gain1/1
  Gain/1 -> Demux2/1
  Gain1/1 -> Demux4/1
  Demux2/1 -> Vx/1, Sum/1
  Demux2/2 -> Vy/1, Sum1/1
  Demux2/3 -> Vz/1, Sum2/1
  Demux4/1 -> wx/1, Sum5/1
  Demux4/2 -> wy/1, Sum4/1
  Demux4/3 -> wz/1, Sum3/1
  In1/1 -> Demux1/1
  Demux5/1 -> Vx1/1, Sum/2
  Demux5/2 -> Vy1/1, Sum1/2
  Demux5/3 -> Vz1/1, Sum2/2
  Demux6/1 -> wx1/1, Sum5/2
  Demux6/2 -> wy1/1, Sum4/2
  Demux6/3 -> wz1/1, Sum3/2
  In2/1 -> Demux3/1
  Sum5/1 -> Vx5/1
  Sum4/1 -> ErrWy/1
  Sum3/1 -> ErrWz/1
  Sum2/1 -> ErrVz/1
  Sum1/1 -> ErrVy/1
  Sum/1 -> ErrVx/1
  Mux/1 -> Demux5/1
  Mux1/1 -> Demux6/1
  Demux3/1 -> Sign1/1
  Demux3/2 -> Sign2/1
  Demux3/3 -> Sign3/1
  Demux3/4 -> Sign4/1
  Demux3/5 -> Sign5/1
  Demux3/6 -> Sign6/1
  Sign1/1 -> Mux/2
  Sign2/1 -> Mux/3
  Sign3/1 -> Mux/1
  Sign4/1 -> Mux1/2
  Sign5/1 -> Mux1/3
  Sign6/1 -> Mux1/1

== system EurlerDynJointVerify/Error Analysis/BodyInfoDisplay/Vel/Jnt4 ==
  note: ErrWx
  In1 : Inport
  In2 : Inport  Port=2
  Demux1 : Demux  Outputs=2
  Demux{2,4..6} (4 alike) : Demux  Outputs=3
  Demux3 : Demux  Outputs=6
  ErrVx : Scope
      settings: TimeRange=10  YMin=-3e-017  YMax=4e-017  SaveName=ScopeData51
  ErrVy : Scope
      settings: TimeRange=10  YMin=-3e-017  YMax=4e-017  SaveName=ScopeData52
  ErrVz : Scope
      settings: TimeRange=10  YMin=-3e-017  YMax=4e-017  SaveName=ScopeData53
  ErrWy : Scope
      settings: TimeRange=10  YMin=-3e-017  YMax=4e-017  SaveName=ScopeData56
  ErrWz : Scope
      settings: TimeRange=10  YMin=-3e-017  YMax=4e-017  SaveName=ScopeData68
  Gain : Gain  Gain=1000
  Gain1 : Gain  Gain=180/pi
  Mux : Mux  Inputs=3
  Mux1 : Mux  Inputs=3
  Sign{1,3..4,6} (4 alike) : Gain
  Sign2 : Gain  Gain=-1
  Sign5 : Gain  Gain=-1
  Sum{,1..5} (6 alike) : Sum  Inputs=-|+
  Vx : Scope
      settings: TimeRange=10  YMin=-3e-017  YMax=4e-017  SaveName=ScopeData40
  Vx1 : Scope
      settings: TimeRange=10  YMin=-3e-017  YMax=4e-017  SaveName=ScopeData45
  Vx5 : Scope
      settings: TimeRange=10  YMin=-3e-017  YMax=4e-017  SaveName=ScopeData54
  Vy : Scope
      settings: TimeRange=10  YMin=-3e-017  YMax=4e-017  SaveName=ScopeData39
  Vy1 : Scope
      settings: TimeRange=10  YMin=-3e-017  YMax=4e-017  SaveName=ScopeData46
  Vz : Scope
      settings: TimeRange=10  YMin=-3e-017  YMax=4e-017  SaveName=ScopeData41
  Vz1 : Scope
      settings: TimeRange=10  YMin=-3e-017  YMax=4e-017  SaveName=ScopeData47
  wx : Scope
      settings: TimeRange=3  YMin=-125  YMax=125  SaveName=ScopeData42
  wx1 : Scope
      settings: TimeRange=3  YMin=-125  YMax=125  SaveName=ScopeData48
  wy : Scope
      settings: TimeRange=10  YMin=-3e-017  YMax=4e-017  SaveName=ScopeData43
  wy1 : Scope
      settings: TimeRange=10  YMin=-3e-017  YMax=4e-017  SaveName=ScopeData49
  wz : Scope
      settings: TimeRange=10  YMin=-3e-017  YMax=4e-017  SaveName=ScopeData44
  wz1 : Scope
      settings: TimeRange=10  YMin=-3e-017  YMax=4e-017  SaveName=ScopeData50
  wires:
  Demux3/6 -> Sign6/1
  Demux3/5 -> Sign5/1
  Demux3/4 -> Sign4/1
  Demux3/3 -> Sign3/1
  Demux3/2 -> Sign2/1
  Demux3/1 -> Sign1/1
  Mux1/1 -> Demux6/1
  Mux/1 -> Demux5/1
  Sum/1 -> ErrVx/1
  Sum1/1 -> ErrVy/1
  Sum2/1 -> ErrVz/1
  Sum3/1 -> ErrWz/1
  Sum4/1 -> ErrWy/1
  Sum5/1 -> Vx5/1
  In2/1 -> Demux3/1
  Demux6/3 -> Sum3/2, wz1/1
  Demux6/2 -> Sum4/2, wy1/1
  Demux6/1 -> Sum5/2, wx1/1
  Demux5/3 -> Sum2/2, Vz1/1
  Demux5/2 -> Sum1/2, Vy1/1
  Demux5/1 -> Sum/2, Vx1/1
  In1/1 -> Demux1/1
  Demux4/3 -> Sum3/1, wz/1
  Demux4/2 -> Sum4/1, wy/1
  Demux4/1 -> Sum5/1, wx/1
  Demux2/3 -> Sum2/1, Vz/1
  Demux2/2 -> Sum1/1, Vy/1
  Demux2/1 -> Sum/1, Vx/1
  Gain1/1 -> Demux4/1
  Gain/1 -> Demux2/1
  Demux1/2 -> Gain1/1
  Demux1/1 -> Gain/1
  Sign1/1 -> Mux/3
  Sign2/1 -> Mux/2
  Sign3/1 -> Mux/1
  Sign4/1 -> Mux1/3
  Sign5/1 -> Mux1/2
  Sign6/1 -> Mux1/1

== system EurlerDynJointVerify/Error Analysis/BodyInfoDisplay/Vel/Jnt5 ==
  note: ErrWx
  In1 : Inport
  In2 : Inport  Port=2
  Demux1 : Demux  Outputs=2
  Demux{2,4..6} (4 alike) : Demux  Outputs=3
  Demux3 : Demux  Outputs=6
  ErrVx : Scope
      settings: TimeRange=10  YMin=-3e-017  YMax=4e-017  SaveName=ScopeData51
  ErrVy : Scope
      settings: TimeRange=10  YMin=-3e-017  YMax=4e-017  SaveName=ScopeData52
  ErrVz : Scope
      settings: TimeRange=10  YMin=-3e-017  YMax=4e-017  SaveName=ScopeData53
  ErrWy : Scope
      settings: TimeRange=10  YMin=-3e-017  YMax=4e-017  SaveName=ScopeData56
  ErrWz : Scope
      settings: TimeRange=10  YMin=-3e-017  YMax=4e-017  SaveName=ScopeData68
  Gain : Gain  Gain=1000
  Gain1 : Gain  Gain=180/pi
  Mux : Mux  Inputs=3
  Mux1 : Mux  Inputs=3
  Sign{1,3..4,6} (4 alike) : Gain  Gain=-1
  Sign2 : Gain
  Sign5 : Gain
  Sum{,1..5} (6 alike) : Sum  Inputs=-|+
  Vx : Scope
      settings: TimeRange=10  YMin=-3e-017  YMax=4e-017  SaveName=ScopeData40
  Vx1 : Scope
      settings: TimeRange=10  YMin=-3e-017  YMax=4e-017  SaveName=ScopeData45
  Vx5 : Scope
      settings: TimeRange=10  YMin=-3e-017  YMax=4e-017  SaveName=ScopeData54
  Vy : Scope
      settings: TimeRange=10  YMin=-3e-017  YMax=4e-017  SaveName=ScopeData39
  Vy1 : Scope
      settings: TimeRange=10  YMin=-3e-017  YMax=4e-017  SaveName=ScopeData46
  Vz : Scope
      settings: TimeRange=10  YMin=-3e-017  YMax=4e-017  SaveName=ScopeData41
  Vz1 : Scope
      settings: TimeRange=10  YMin=-3e-017  YMax=4e-017  SaveName=ScopeData47
  wx : Scope
      settings: TimeRange=3  YMin=-125  YMax=125  SaveName=ScopeData42
  wx1 : Scope
      settings: TimeRange=3  YMin=-125  YMax=125  SaveName=ScopeData48
  wy : Scope
      settings: TimeRange=10  YMin=-3e-017  YMax=4e-017  SaveName=ScopeData43
  wy1 : Scope
      settings: TimeRange=10  YMin=-3e-017  YMax=4e-017  SaveName=ScopeData49
  wz : Scope
      settings: TimeRange=10  YMin=-3e-017  YMax=4e-017  SaveName=ScopeData44
  wz1 : Scope
      settings: TimeRange=10  YMin=-3e-017  YMax=4e-017  SaveName=ScopeData50
  wires:
  Demux1/1 -> Gain/1
  Demux1/2 -> Gain1/1
  Gain/1 -> Demux2/1
  Gain1/1 -> Demux4/1
  Demux2/1 -> Vx/1, Sum/1
  Demux2/2 -> Vy/1, Sum1/1
  Demux2/3 -> Vz/1, Sum2/1
  Demux4/1 -> wx/1, Sum5/1
  Demux4/2 -> wy/1, Sum4/1
  Demux4/3 -> wz/1, Sum3/1
  In1/1 -> Demux1/1
  Demux5/1 -> Vx1/1, Sum/2
  Demux5/2 -> Vy1/1, Sum1/2
  Demux5/3 -> Vz1/1, Sum2/2
  Demux6/1 -> wx1/1, Sum5/2
  Demux6/2 -> wy1/1, Sum4/2
  Demux6/3 -> wz1/1, Sum3/2
  In2/1 -> Demux3/1
  Sum5/1 -> Vx5/1
  Sum4/1 -> ErrWy/1
  Sum3/1 -> ErrWz/1
  Sum2/1 -> ErrVz/1
  Sum1/1 -> ErrVy/1
  Sum/1 -> ErrVx/1
  Mux/1 -> Demux5/1
  Mux1/1 -> Demux6/1
  Demux3/1 -> Sign1/1
  Demux3/2 -> Sign2/1
  Demux3/3 -> Sign3/1
  Demux3/4 -> Sign4/1
  Demux3/5 -> Sign5/1
  Demux3/6 -> Sign6/1
  Sign1/1 -> Mux/2
  Sign2/1 -> Mux/3
  Sign3/1 -> Mux/1
  Sign4/1 -> Mux1/2
  Sign5/1 -> Mux1/3
  Sign6/1 -> Mux1/1

== system EurlerDynJointVerify/Error Analysis/BodyInfoDisplay/Vel/Jnt6 ==
  note: ErrWx
  In1 : Inport
  In2 : Inport  Port=2
  Demux1 : Demux  Outputs=2
  Demux{2,4..6} (4 alike) : Demux  Outputs=3
  Demux3 : Demux  Outputs=6
  ErrVx : Scope
      settings: TimeRange=10  YMin=-3e-017  YMax=4e-017  SaveName=ScopeData51
  ErrVy : Scope
      settings: TimeRange=10  YMin=-3e-017  YMax=4e-017  SaveName=ScopeData52
  ErrVz : Scope
      settings: TimeRange=10  YMin=-3e-017  YMax=4e-017  SaveName=ScopeData53
  ErrWy : Scope
      settings: TimeRange=10  YMin=-3e-017  YMax=4e-017  SaveName=ScopeData56
  ErrWz : Scope
      settings: TimeRange=10  YMin=-3e-017  YMax=4e-017  SaveName=ScopeData68
  Gain : Gain  Gain=1000
  Gain1 : Gain  Gain=180/pi
  Mux : Mux  Inputs=3
  Mux1 : Mux  Inputs=3
  Sign{1,3..4,6} (4 alike) : Gain
  Sign2 : Gain  Gain=-1
  Sign5 : Gain  Gain=-1
  Sum{,1..5} (6 alike) : Sum  Inputs=-|+
  Vx : Scope
      settings: TimeRange=10  YMin=-3e-017  YMax=4e-017  SaveName=ScopeData40
  Vx1 : Scope
      settings: TimeRange=10  YMin=-3e-017  YMax=4e-017  SaveName=ScopeData45
  Vx5 : Scope
      settings: TimeRange=10  YMin=-3e-017  YMax=4e-017  SaveName=ScopeData54
  Vy : Scope
      settings: TimeRange=10  YMin=-3e-017  YMax=4e-017  SaveName=ScopeData39
  Vy1 : Scope
      settings: TimeRange=10  YMin=-3e-017  YMax=4e-017  SaveName=ScopeData46
  Vz : Scope
      settings: TimeRange=10  YMin=-3e-017  YMax=4e-017  SaveName=ScopeData41
  Vz1 : Scope
      settings: TimeRange=10  YMin=-3e-017  YMax=4e-017  SaveName=ScopeData47
  wx : Scope
      settings: TimeRange=3  YMin=-125  YMax=125  SaveName=ScopeData42
  wx1 : Scope
      settings: TimeRange=3  YMin=-125  YMax=125  SaveName=ScopeData48
  wy : Scope
      settings: TimeRange=10  YMin=-3e-017  YMax=4e-017  SaveName=ScopeData43
  wy1 : Scope
      settings: TimeRange=10  YMin=-3e-017  YMax=4e-017  SaveName=ScopeData49
  wz : Scope
      settings: TimeRange=10  YMin=-3e-017  YMax=4e-017  SaveName=ScopeData44
  wz1 : Scope
      settings: TimeRange=10  YMin=-3e-017  YMax=4e-017  SaveName=ScopeData50
  wires:
  Demux3/6 -> Sign6/1
  Demux3/5 -> Sign5/1
  Demux3/4 -> Sign4/1
  Demux3/3 -> Sign3/1
  Demux3/2 -> Sign2/1
  Demux3/1 -> Sign1/1
  Mux1/1 -> Demux6/1
  Mux/1 -> Demux5/1
  Sum/1 -> ErrVx/1
  Sum1/1 -> ErrVy/1
  Sum2/1 -> ErrVz/1
  Sum3/1 -> ErrWz/1
  Sum4/1 -> ErrWy/1
  Sum5/1 -> Vx5/1
  In2/1 -> Demux3/1
  Demux6/3 -> Sum3/2, wz1/1
  Demux6/2 -> Sum4/2, wy1/1
  Demux6/1 -> Sum5/2, wx1/1
  Demux5/3 -> Sum2/2, Vz1/1
  Demux5/2 -> Sum1/2, Vy1/1
  Demux5/1 -> Sum/2, Vx1/1
  In1/1 -> Demux1/1
  Demux4/3 -> Sum3/1, wz/1
  Demux4/2 -> Sum4/1, wy/1
  Demux4/1 -> Sum5/1, wx/1
  Demux2/3 -> Sum2/1, Vz/1
  Demux2/2 -> Sum1/1, Vy/1
  Demux2/1 -> Sum/1, Vx/1
  Gain1/1 -> Demux4/1
  Gain/1 -> Demux2/1
  Demux1/2 -> Gain1/1
  Demux1/1 -> Gain/1
  Sign1/1 -> Mux/3
  Sign2/1 -> Mux/2
  Sign3/1 -> Mux/1
  Sign4/1 -> Mux1/3
  Sign5/1 -> Mux1/2
  Sign6/1 -> Mux1/1

== matlab function Circle_XY/Jacobian ==
  data: Omega output double; EndVel input double; Theta input double; L parameter double
function Omega = fcn(EndVel,Theta,L)
%#eml

Omega = zeros(6,1);
V = [EndVel; 0; 0; 0];   
g = fwd_kin(L,Theta');
Jb = body_Jacobian(L,Theta');
Adg_inv = double(AdjointInv(g));
Omega = double((Jb \ Adg_inv* V)')';

== matlab function Circle_XY/Inverse Kinematic ==
  data: EndPos input double; init_Rot parameter double; theta output double; L parameter double
function theta = fcn(EndPos,init_Rot,L)
%#eml
theta =[0;0; 0; 0; 0; 0];
gd = [init_Rot,EndPos;[0 0 0],1];
[theta_total,num_total] = inv_kin(gd,L);
theta = theta_total(:,2);

== matlab function Dynamic Euler/Newton Euler Recursion ==
  data: Pos input double; Torque output double; Vel input double; Acc input double; DH_EU parameter double; Ma_EU parameter double; Cen_EU parameter double; Ie_EU parameter double; Ft_EU parameter double; JntVel output double; JntAcc output double; JntF output double
function [Torque,JntVel,JntAcc,JntF] = fcn(Pos,Vel,Acc,DH_EU,Ma_EU,Cen_EU,Ie_EU,Ft_EU)
%#eml
Torque = [0;0;0;0;0;0];
JntVel = zeros(36,1);
JntAcc = zeros(36,1);
JntF = zeros(36,1);
[Torque,JntVel,JntAcc,JntF] = DynEuler(DH_EU,Ma_EU,Cen_EU,Ie_EU,Ft_EU,Pos,Vel,Acc);
%[Torque,JntVel,JntAcc,JntF] = DynEulerSci(DH_EU,Ma_EU,Cen_EU,Ie_EU,Ft_EU,Pos,Vel,Acc);

== matlab function Circle_XZ/Inverse Kinematic ==
  data: EndPos input double; init_Rot parameter double; theta output double; L parameter double
function theta = fcn(EndPos,init_Rot,L)
%#eml
theta =[0;0; 0; 0; 0; 0];
gd = [init_Rot,EndPos;[0 0 0],1];
[theta_total,num_total] = inv_kin(gd,L);
theta = theta_total(:,2);

== matlab function Circle_XZ/Jacobian ==
  data: Omega output double; EndVel input double; Theta input double; L parameter double
function Omega = fcn(EndVel,Theta,L)
%#eml

Omega = zeros(6,1);
V = [EndVel; 0; 0; 0];   
g = fwd_kin(L,Theta');
Jb = body_Jacobian(L,Theta');
Adg_inv = double(AdjointInv(g));
Omega = double((Jb \ Adg_inv* V)')';

== matlab function Line_A23/Forward ==
  data: Theta input double; EndPos output double; L parameter double
function EndPos = fcn(Theta,L)
%#eml
gd = fwd_kin(L,Theta');
EndPos = gd(1:3,4);

== matlab function Line_A23/Jacobian ==
  data: Theta input double; Omega input double; EndVel output double; L parameter double
function EndVel = fcn(Theta,Omega,L)
%#eml


EndVW = spat_Jacobian(L,Theta')*Omega;
gd = fwd_kin(L,Theta');
EndW = EndVW(4:6,1);
gd_pos = gd(1:3,4);
EndVel=cross(EndW,gd_pos);

== matlab function Line_Acc/Inverse Kinematic ==
  data: EndPos input double; init_Rot parameter double; theta output double; L parameter double
function theta = fcn(EndPos,init_Rot,L)
%#eml
theta =[0;0; 0; 0; 0; 0];
gd = [init_Rot,EndPos;[0 0 0],1];
[theta_total,num_total] = inv_kin(gd,L);
theta = theta_total(:,2);

== matlab function Line_Acc/Jacobian ==
  data: Omega output double; EndVel input double; Theta input double; L parameter double
function Omega = fcn(EndVel,Theta,L)
%#eml

Omega = zeros(6,1);
V = [EndVel; 0; 0; 0];   
g = fwd_kin(L,Theta');
Jb = body_Jacobian(L,Theta');
Adg_inv = double(AdjointInv(g));
Omega = double((Jb \ Adg_inv* V)')';

== matlab function Circle_YZ/Inverse Kinematic ==
  data: EndPos input double; init_Rot parameter double; theta output double; L parameter double
function theta = fcn(EndPos,init_Rot,L)
%#eml
theta =[0;0; 0; 0; 0; 0];
gd = [init_Rot,EndPos;[0 0 0],1];
[theta_total,num_total] = inv_kin(gd,L);
theta = theta_total(:,2);

== matlab function Circle_YZ/Jacobian ==
  data: Omega output double; EndVel input double; Theta input double; L parameter double
function Omega = fcn(EndVel,Theta,L)
%#eml

Omega = zeros(6,1);
V = [EndVel; 0; 0; 0];   
g = fwd_kin(L,Theta');
Jb = body_Jacobian(L,Theta');
Adg_inv = double(AdjointInv(g));
Omega = double((Jb \ Adg_inv* V)')';

== matlab function Line_JointSpace/Forward ==
  data: Theta input double; EndPos output double; L parameter double
function EndPos = fcn(Theta,L)
%#eml
gd = fwd_kin(L,Theta');
EndPos = gd(1:3,4);

== matlab function Line_JointSpace/Jacobian ==
  data: Theta input double; Omega input double; EndVel output double; L parameter double
function EndVel = fcn(Theta,Omega,L)
%#eml


EndVW = spat_Jacobian(L,Theta')*Omega;
gd = fwd_kin(L,Theta');
EndW = EndVW(4:6,1);
gd_pos = gd(1:3,4);
EndVel=cross(EndW,gd_pos);

== matlab function Still/Inverse Kinematic ==
  data: EndPos input double; init_Rot parameter double; theta output double; L parameter double
function theta = fcn(EndPos,init_Rot,L)
%#eml
theta =[0;0; 0; 0; 0; 0];
gd = [init_Rot,EndPos;[0 0 0],1];
[theta_total,num_total] = inv_kin(gd,L);
theta = theta_total(:,2);

== matlab function Still/Jacobian ==
  data: Omega output double; EndVel input double; Theta input double; L parameter double
function Omega = fcn(EndVel,Theta,L)
%#eml

Omega = zeros(6,1);
V = [EndVel; 0; 0; 0];   
g = fwd_kin(L,Theta');
Jb = body_Jacobian(L,Theta');
Adg_inv = double(AdjointInv(g));
Omega = double((Jb \ Adg_inv* V)')';

== matlab function Line/Inverse Kinematic ==
  data: EndPos input double; init_Rot parameter double; theta output double; L parameter double
function theta = fcn(EndPos,init_Rot,L)
%#eml
theta =[0;0; 0; 0; 0; 0];
gd = [init_Rot,EndPos;[0 0 0],1];
[theta_total,num_total] = inv_kin(gd,L);
theta = theta_total(:,2);

== matlab function Line/Jacobian ==
  data: Omega output double; EndVel input double; Theta input double; L parameter double
function Omega = fcn(EndVel,Theta,L)
%#eml

Omega = zeros(6,1);
V = [EndVel; 0; 0; 0];   
g = fwd_kin(L,Theta');
Jb = body_Jacobian(L,Theta');
Adg_inv = double(AdjointInv(g));
Omega = double((Jb \ Adg_inv* V)')';

== matlab function Joint/Forward ==
  data: Theta input double; EndPos output double; L parameter double
function EndPos = fcn(Theta,L)
%#eml
gd = fwd_kin(L,Theta');
EndPos = gd(1:3,4);

== matlab function Joint/Jacobian ==
  data: Theta input double; Omega input double; EndVel output double; L parameter double
function EndVel = fcn(Theta,Omega,L)
%#eml


EndVW = spat_Jacobian(L,Theta')*Omega;
gd = fwd_kin(L,Theta');
EndW = EndVW(4:6,1);
gd_pos = gd(1:3,4);
EndVel=cross(EndW,gd_pos);

== matlab function Dynamic Euler/Newton Euler Recursion Min ==
  data: Pos input double; Torque output double; Vel input double; Acc input double; DH_Min parameter double; Ma_Min parameter double; Cen_Min parameter double; Ie_Min parameter double; Ft_Min parameter double; JntVel output double; JntAcc output double; JntF output double
function [Torque,JntVel,JntAcc,JntF] = fcn(Pos,Vel,Acc,DH_Min,Ma_Min, Cen_Min, Ie_Min, Ft_Min)
%#eml
Torque = [0;0;0;0;0;0];
JntVel = zeros(36,1);
JntAcc = zeros(36,1);
JntF = zeros(36,1);
[Torque,JntVel,JntAcc,JntF] = DynEuler_Min(DH_Min,Ma_Min,Cen_Min,Ie_Min,Ft_Min,Pos,Vel,Acc);
%[Torque,JntVel,JntAcc,JntF] = DynEulerSci(DH_EU,Ma_EU,Cen_EU,Ie_EU,Ft_EU,Pos,Vel,Acc);
